simulink model "mpu6050 - Copy"  (R2017a)
settings: Solver=FixedStepDiscrete  StartTime=0.0  StopTime=inf  RelTol=1e-3
PostLoadFcn:
  | ChipSelect = 1;  % choose I2C comms
  | AddressAlt = 0;  % use default address
  | 
  | if AddressAlt == 1
  | % b1101001 (pin AD0 is logic high).
  | SlvAddr = uint8(bin2dec('1101001'));  % ADDR ALT = 1
  | else
  | % b1101000 (pin AD0 is logic low)
  | SlvAddr = uint8(bin2dec('1101000'));  % ADDR ALT = 0
  | end
  | SlvAddr = uint8(hex2dec('68'));
  | 
  | 
  | % 0x3B 59 ACCEL_XOUT[15:8]
  | % 0x3C 60 ACCEL_XOUT[7:0]
  | % 0x3D 61 ACCEL_YOUT[15:8]
  | % 0x3E 62 ACCEL_YOUT[7:0]
  | % 0x3F 63 ACCEL_ZOUT[15:8]
  | % 0x40 64 ACCEL_ZOUT[7:0]
  | 
  | AccelXRegAddr = uint8(hex2dec('3B'));
  | AccelYRegAddr = uint8(hex2dec('3D'));
  | AccelZRegAddr = uint8(hex2dec('3F'));
  | 
  | % 0x43 67 GYRO_XOUT[15:8]
  | % 0x44 68 GYRO_XOUT[7:0]
  | % 0x45 69 GYRO_YOUT[15:8]
  | % 0x46 70 GYRO_YOUT[7:0]
  | % 0x47 71 GYRO_ZOUT[15:8]
  | % 0x48 72 GYRO_ZOUT[7:0]
  | 
  | GyroXRegAddr = uint8(hex2dec('43'));
  | GyroYRegAddr = uint8(hex2dec('45'));
  | GyroZRegAddr = uint8(hex2dec('47'));
  | 
  | deviceAddr = fi(SlvAddr,0,7,0);
  | 
  | powerRegAddr = uint8(hex2dec('6B'));
  | powerRegData = bin2dec('10000001');
(part 1 of 4)
settings Model: DataTypeOverride=Off  Creator=skuznick  LastModifiedBy=mini
settings DataIOCC: SaveOutput=off  SaveTime=off
settings OptimizationCC: BlockReduction=off  ConditionallyExecuteInputs=off  DefaultParameterBehavior=Inlined
settings DebuggingCC: AlgebraicLoopMsg=error  SingleTaskRateTransMsg=error
settings HardwareCC: ProdBitPerPointer=32  ProdBitPerSizeT=32  ProdBitPerPtrDiffT=32  ProdLargestAtomicFloat=None  ProdIntDivRoundTo=Undefined  ProdEndianess=Unspecified  ProdWordSize=32  ProdHWDeviceType=ASIC/FPGA->ASIC/FPGA  ProdEqTarget=off
settings GRTTargetCC: ExtMode=on

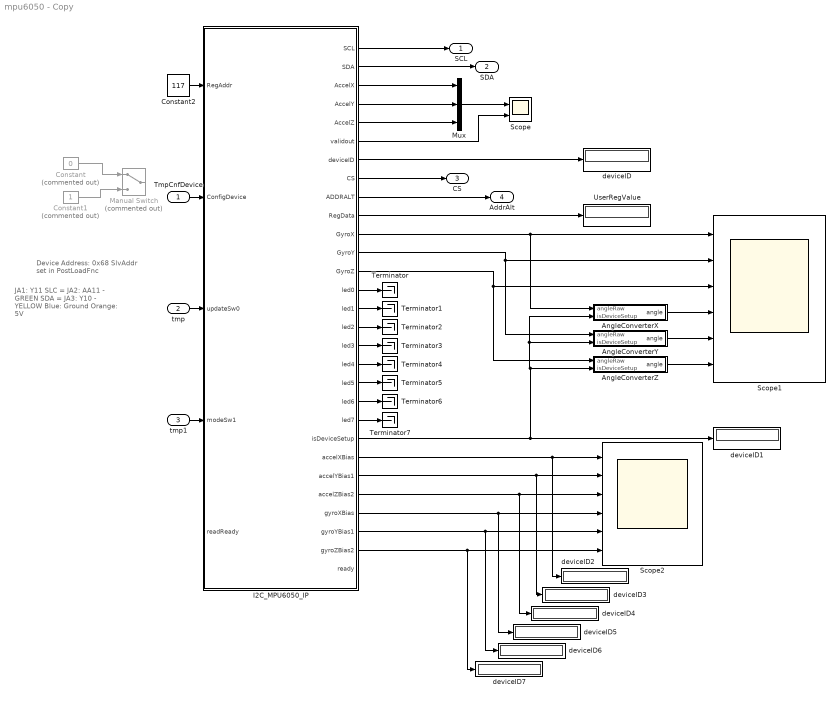
== system mpu6050 - Copy ==
  note: JA1: Y11
      | SLC = JA2: AA11 - GREEN
      | SDA = JA3: Y10  - YELLOW
      | Blue: Ground
      | Orange: 5V
  note: Device Address: 0x68
      | SlvAddr set in PostLoadFnc
  TmpCnfDevice : Inport  OutDataTypeStr=boolean
  tmp : Inport  Port=2  OutDataTypeStr=boolean
  tmp1 : Inport  Port=3  OutDataTypeStr=boolean
  AngleConverterX : Subsystem
  AngleConverterY : Subsystem
  AngleConverterZ : Subsystem
  Constant : Constant  Commented=on  Value=0  OutDataTypeStr=boolean  SampleTime=-1
  Constant1 : Constant  Commented=on  OutDataTypeStr=boolean  SampleTime=-1
  Constant2 : Constant  Value=117  OutDataTypeStr=uint8  SampleTime=-1
  I2C_MPU6050_IP : Subsystem  TreatAsAtomicUnit=on  SystemSampleTime=1/400e3
  Manual Switch : ManualSwitch  Commented=on
  Mux : Mux  Inputs=3
  Scope : Scope  NumInputPorts=2
  Scope1 : Scope  NumInputPorts=6
  Scope2 : Scope  NumInputPorts=6
  Terminator{,1..7} (8 alike) : Terminator
  UserRegValue : Display
  deviceID{,1..7} (8 alike) : Display
      deviceID2 settings: Decimation=5
      deviceID3 settings: Decimation=5
      deviceID4 settings: Decimation=5
      deviceID5 settings: Decimation=5
      deviceID6 settings: Decimation=5
      deviceID7 settings: Decimation=5
  SCL : Outport
  SDA : Outport  Port=2
  CS : Outport  Port=3
  AddrAlt : Outport  Port=4
  wires:
  I2C_MPU6050_IP/2(SDA) -> SDA/1
  I2C_MPU6050_IP/1(SCL) -> SCL/1
  I2C_MPU6050_IP/8(CS) -> CS/1
  I2C_MPU6050_IP/9(ADDRALT) -> AddrAlt/1
  I2C_MPU6050_IP/4(AccelY) -> Mux/2
  I2C_MPU6050_IP/3(AccelX) -> Mux/1
  I2C_MPU6050_IP/5(AccelZ) -> Mux/3
  I2C_MPU6050_IP/7(deviceID) -> deviceID/1
  I2C_MPU6050_IP/10(RegData) -> UserRegValue/1
  Mux/1 -> Scope/1
  Constant/1 -> Manual Switch/1
  Constant1/1 -> Manual Switch/2
  Constant2/1 -> I2C_MPU6050_IP/1(RegAddr)
  I2C_MPU6050_IP/13(GyroZ) -> AngleConverterZ/1(angleRaw), Scope1/3
  I2C_MPU6050_IP/11(GyroX) -> AngleConverterX/1(angleRaw), Scope1/1
  I2C_MPU6050_IP/12(GyroY) -> AngleConverterY/1(angleRaw), Scope1/2
  I2C_MPU6050_IP/6(validout) -> Scope/2
  TmpCnfDevice/1 -> I2C_MPU6050_IP/2(ConfigDevice)
  I2C_MPU6050_IP/14(led0) -> Terminator/1
  I2C_MPU6050_IP/15(led1) -> Terminator1/1
  I2C_MPU6050_IP/16(led2) -> Terminator2/1
  I2C_MPU6050_IP/17(led3) -> Terminator3/1
  I2C_MPU6050_IP/20(led6) -> Terminator6/1
  I2C_MPU6050_IP/21(led7) -> Terminator7/1
  I2C_MPU6050_IP/19(led5) -> Terminator5/1
  I2C_MPU6050_IP/18(led4) -> Terminator4/1
  tmp/1 -> I2C_MPU6050_IP/3(updateSw0)
  tmp1/1 -> I2C_MPU6050_IP/4(modeSw1)
  I2C_MPU6050_IP/22(isDeviceSetup) -> deviceID1/1, AngleConverterZ/2(isDeviceSetup), AngleConverterX/2(isDeviceSetup), AngleConverterY/2(isDeviceSetup)
  AngleConverterY/1(angle) -> Scope1/5
  AngleConverterZ/1(angle) -> Scope1/6
  AngleConverterX/1(angle) -> Scope1/4
  I2C_MPU6050_IP/23(accelXBias) -> deviceID2/1, Scope2/1
  I2C_MPU6050_IP/24(accelYBias1) -> deviceID3/1, Scope2/2
  I2C_MPU6050_IP/25(accelZBias2) -> deviceID4/1, Scope2/3
  I2C_MPU6050_IP/26(gyroXBias) -> deviceID5/1, Scope2/4
  I2C_MPU6050_IP/27(gyroYBias1) -> deviceID6/1, Scope2/5
  I2C_MPU6050_IP/28(gyroZBias2) -> deviceID7/1, Scope2/6

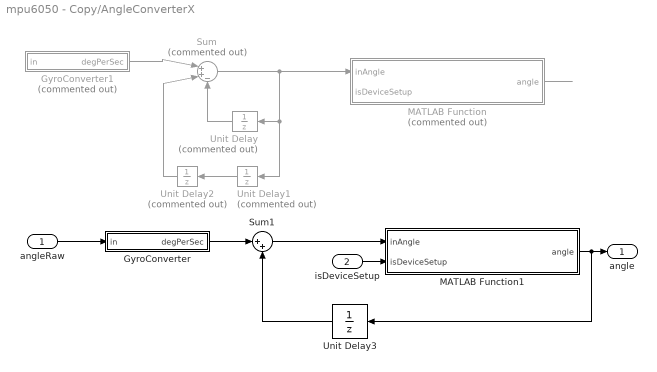
== system mpu6050 - Copy/AngleConverterX ==
  angleRaw : Inport  OutDataTypeStr=int16  Interpolate=off
  isDeviceSetup : Inport  Port=2  OutDataTypeStr=boolean  Interpolate=off
  GyroConverter : Subsystem
  GyroConverter1 : Subsystem  Commented=on
  MATLAB Function : MATLAB Function  Commented=on  TreatAsAtomicUnit=on
  MATLAB Function1 : MATLAB Function  TreatAsAtomicUnit=on
  Sum : Sum  Commented=on  Inputs=|++-  SaturateOnIntegerOverflow=off  InputSameDT=off  OutDataTypeStr=Inherit: Inherit via internal rule
  Sum1 : Sum  Inputs=|++  SaturateOnIntegerOverflow=off  InputSameDT=off  OutDataTypeStr=Inherit: Inherit via internal rule
  Unit Delay : UnitDelay  Commented=on  SampleTime=-1
  Unit Delay1 : UnitDelay  Commented=on  SampleTime=-1
  Unit Delay2 : UnitDelay  Commented=on  SampleTime=-1
  Unit Delay3 : UnitDelay  SampleTime=-1
  angle : Outport  OutDataTypeStr=double
  wires:
  Sum/1 -> Unit Delay1/1, Unit Delay/1, MATLAB Function/1(inAngle)
  GyroConverter1/1(degPerSec) -> Sum/1
  Unit Delay/1 -> Sum/3
  Unit Delay1/1 -> Unit Delay2/1
  Unit Delay2/1 -> Sum/2
  MATLAB Function/1(angle) -> ?
  ? -> MATLAB Function/2(isDeviceSetup)
  MATLAB Function1/1(angle) -> Unit Delay3/1, angle/1
  angleRaw/1 -> GyroConverter/1(in)
  isDeviceSetup/1 -> MATLAB Function1/2(isDeviceSetup)
  GyroConverter/1(degPerSec) -> Sum1/1
  Sum1/1 -> MATLAB Function1/1(inAngle)
  Unit Delay3/1 -> Sum1/2

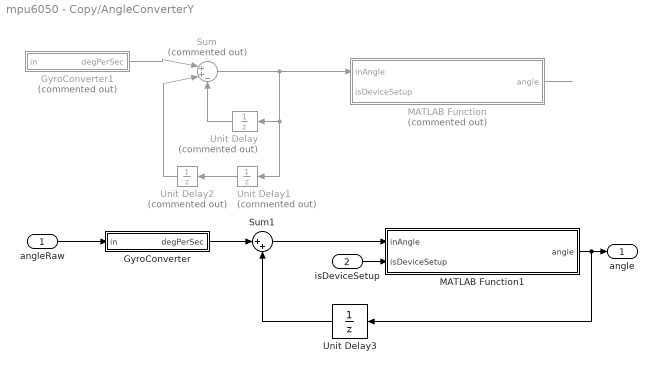
== system mpu6050 - Copy/AngleConverterY ==
  angleRaw : Inport  OutDataTypeStr=int16  Interpolate=off
  isDeviceSetup : Inport  Port=2  OutDataTypeStr=boolean  Interpolate=off
  GyroConverter : Subsystem
  GyroConverter1 : Subsystem  Commented=on
  MATLAB Function : MATLAB Function  Commented=on  TreatAsAtomicUnit=on
  MATLAB Function1 : MATLAB Function  TreatAsAtomicUnit=on
  Sum : Sum  Commented=on  Inputs=|++-  SaturateOnIntegerOverflow=off  InputSameDT=off  OutDataTypeStr=Inherit: Inherit via internal rule
  Sum1 : Sum  Inputs=|++  SaturateOnIntegerOverflow=off  InputSameDT=off  OutDataTypeStr=Inherit: Inherit via internal rule
  Unit Delay : UnitDelay  Commented=on  SampleTime=-1
  Unit Delay1 : UnitDelay  Commented=on  SampleTime=-1
  Unit Delay2 : UnitDelay  Commented=on  SampleTime=-1
  Unit Delay3 : UnitDelay  SampleTime=-1
  angle : Outport  OutDataTypeStr=double
  wires:
  Sum/1 -> Unit Delay1/1, Unit Delay/1, MATLAB Function/1(inAngle)
  GyroConverter1/1(degPerSec) -> Sum/1
  Unit Delay/1 -> Sum/3
  Unit Delay1/1 -> Unit Delay2/1
  Unit Delay2/1 -> Sum/2
  MATLAB Function/1(angle) -> ?
  ? -> MATLAB Function/2(isDeviceSetup)
  MATLAB Function1/1(angle) -> Unit Delay3/1, angle/1
  angleRaw/1 -> GyroConverter/1(in)
  isDeviceSetup/1 -> MATLAB Function1/2(isDeviceSetup)
  GyroConverter/1(degPerSec) -> Sum1/1
  Sum1/1 -> MATLAB Function1/1(inAngle)
  Unit Delay3/1 -> Sum1/2

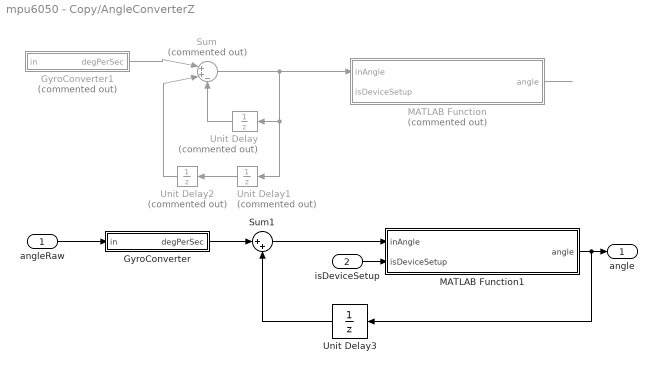
== system mpu6050 - Copy/AngleConverterZ ==
  angleRaw : Inport  OutDataTypeStr=int16  Interpolate=off
  isDeviceSetup : Inport  Port=2  OutDataTypeStr=boolean  Interpolate=off
  GyroConverter : Subsystem
  GyroConverter1 : Subsystem  Commented=on
  MATLAB Function : MATLAB Function  Commented=on  TreatAsAtomicUnit=on
  MATLAB Function1 : MATLAB Function  TreatAsAtomicUnit=on
  Sum : Sum  Commented=on  Inputs=|++-  SaturateOnIntegerOverflow=off  InputSameDT=off  OutDataTypeStr=Inherit: Inherit via internal rule
  Sum1 : Sum  Inputs=|++  SaturateOnIntegerOverflow=off  InputSameDT=off  OutDataTypeStr=Inherit: Inherit via internal rule
  Unit Delay : UnitDelay  Commented=on  SampleTime=-1
  Unit Delay1 : UnitDelay  Commented=on  SampleTime=-1
  Unit Delay2 : UnitDelay  Commented=on  SampleTime=-1
  Unit Delay3 : UnitDelay  SampleTime=-1
  angle : Outport  OutDataTypeStr=double
  wires:
  Sum/1 -> Unit Delay1/1, Unit Delay/1, MATLAB Function/1(inAngle)
  GyroConverter1/1(degPerSec) -> Sum/1
  Unit Delay/1 -> Sum/3
  Unit Delay1/1 -> Unit Delay2/1
  Unit Delay2/1 -> Sum/2
  MATLAB Function/1(angle) -> ?
  ? -> MATLAB Function/2(isDeviceSetup)
  MATLAB Function1/1(angle) -> Unit Delay3/1, angle/1
  angleRaw/1 -> GyroConverter/1(in)
  isDeviceSetup/1 -> MATLAB Function1/2(isDeviceSetup)
  GyroConverter/1(degPerSec) -> Sum1/1
  Sum1/1 -> MATLAB Function1/1(inAngle)
  Unit Delay3/1 -> Sum1/2

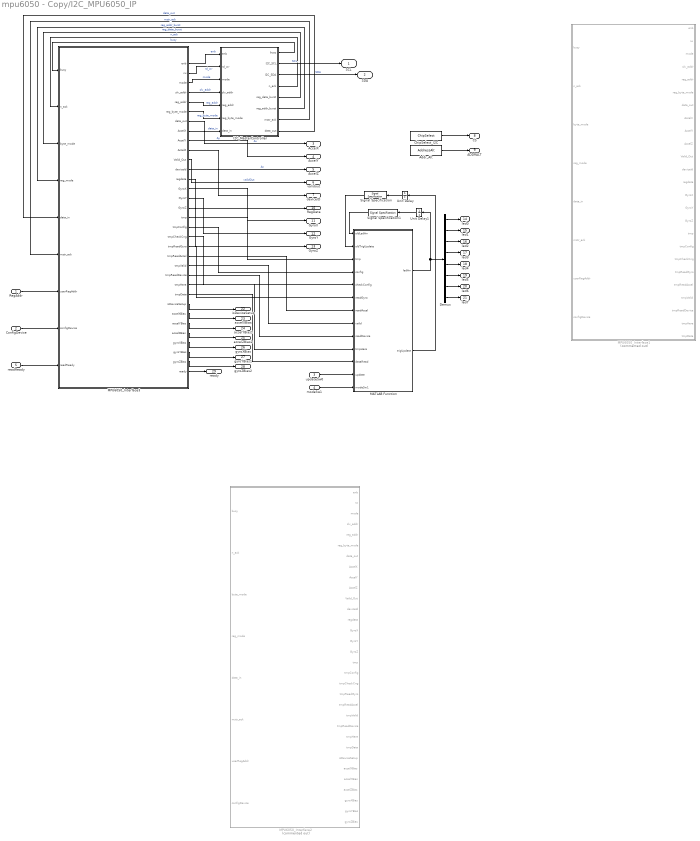
== system mpu6050 - Copy/I2C_MPU6050_IP ==
  RegAddr : Inport
  ConfigDevice : Inport  Port=2
  updateSw0 : Inport  Port=3  OutDataTypeStr=boolean
  modeSw1 : Inport  Port=4  OutDataTypeStr=boolean
  readReady : Inport  Port=5
  Addr_Alt : Constant  Value=AddressAlt  OutDataTypeStr=boolean  SampleTime=-1
  ChipSelect_I2C : Constant  Value=ChipSelect  OutDataTypeStr=boolean  SampleTime=-1
  Demux : Demux  Outputs=8
  I2C_MasterController : Subsystem
  MATLAB Function : MATLAB Function  TreatAsAtomicUnit=on
  MPU6050_Interface1 : Stateflow chart  Commented=on  TreatAsAtomicUnit=on
  MPU6050_Interface2 : Stateflow chart  Commented=on  TreatAsAtomicUnit=on
  MPU6050_Interface3 : Stateflow chart  TreatAsAtomicUnit=on
  Signal Specification : SignalSpecification  OutDataTypeStr=boolean
  Signal Specification1 : SignalSpecification  OutDataTypeStr=boolean  Dimensions=[1 8]
  Unit Delay : UnitDelay  SampleTime=-1
  Unit Delay1 : UnitDelay  SampleTime=-1
  SCL : Outport
  SDA : Outport  Port=2
  AccelX : Outport  Port=3
  AccelY : Outport  Port=4
  AccelZ : Outport  Port=5
  validout : Outport  Port=6
  deviceID : Outport  Port=7
  CS : Outport  Port=8
  ADDRALT : Outport  Port=9
  RegData : Outport  Port=10
  GyroX : Outport  Port=11
  GyroY : Outport  Port=12
  GyroZ : Outport  Port=13
  led0 : Outport  Port=14  OutDataTypeStr=boolean
  led1 : Outport  Port=15  OutDataTypeStr=boolean
  led2 : Outport  Port=16  OutDataTypeStr=boolean
  led3 : Outport  Port=17  OutDataTypeStr=boolean
  led4 : Outport  Port=18  OutDataTypeStr=boolean
  led5 : Outport  Port=19  OutDataTypeStr=boolean
  led6 : Outport  Port=20  OutDataTypeStr=boolean
  led7 : Outport  Port=21  OutDataTypeStr=boolean
  isDeviceSetup : Outport  Port=22  OutDataTypeStr=boolean
  accelXBias : Outport  Port=23
  accelYBias1 : Outport  Port=24
  accelZBias2 : Outport  Port=25
  gyroXBias : Outport  Port=26
  gyroYBias1 : Outport  Port=27
  gyroZBias2 : Outport  Port=28
  ready : Outport  Port=29  OutDataTypeStr=boolean
  wires:
  MPU6050_Interface3/7(data_out) -> I2C_MasterController/7(data_in)  "data_in"
  I2C_MasterController/8(data_out) -> MPU6050_Interface3/5(data_in)  "data_out"
  I2C_MasterController/7(mstr_ack) -> MPU6050_Interface3/6(mstr_ack)  "mstr_ack"
  I2C_MasterController/4(n_ack) -> MPU6050_Interface3/2(n_ack)  "n_ack"
  I2C_MasterController/5(reg_data_burst) -> MPU6050_Interface3/3(byte_mode)  "reg_data_burst"
  I2C_MasterController/6(reg_addr_burst) -> MPU6050_Interface3/4(reg_mode)  "reg_addr_burst"
  I2C_MasterController/1(busy) -> MPU6050_Interface3/1(busy)  "busy"
  I2C_MasterController/3(I2C_SDA) -> SDA/1  "SDA"
  I2C_MasterController/2(I2C_SCL) -> SCL/1  "SCL"
  MPU6050_Interface3/6(reg_byte_mode) -> I2C_MasterController/6(reg_byte_mode)  "reg_byte_mode"
  MPU6050_Interface3/5(reg_addr) -> I2C_MasterController/5(reg_addr)  "reg_addr"
  MPU6050_Interface3/4(slv_addr) -> I2C_MasterController/4(slv_addr)  "slv_addr"
  MPU6050_Interface3/3(mode) -> I2C_MasterController/3(mode)  "mode"
  MPU6050_Interface3/2(rw) -> I2C_MasterController/2(rd_wr)  "rd_wr"
  MPU6050_Interface3/1(enb) -> I2C_MasterController/1(enb)  "enb"
  ChipSelect_I2C/1 -> CS/1
  Addr_Alt/1 -> ADDRALT/1
  MPU6050_Interface3/9(AccelY) -> AccelY/1  "Ay"
  MPU6050_Interface3/10(AccelZ) -> AccelZ/1  "Az"
  MPU6050_Interface3/11(Valid_Out) -> validout/1  "validOut"
  MPU6050_Interface3/8(AccelX) -> AccelX/1  "Ax"
  MPU6050_Interface3/12(deviceId) -> deviceID/1
  MPU6050_Interface3/13(regdata) -> RegData/1
  RegAddr/1 -> MPU6050_Interface3/7(userRegAddr)
  MPU6050_Interface3/14(GyroX) -> GyroX/1
  MPU6050_Interface3/15(GyroY) -> GyroY/1
  MPU6050_Interface3/16(GyroZ) -> GyroZ/1
  ConfigDevice/1 -> MPU6050_Interface3/8(configDevice)
  MPU6050_Interface3/17(tmp) -> MATLAB Function/3(tmp)
  MPU6050_Interface3/18(tmpConfig) -> MATLAB Function/4(config)
  MPU6050_Interface3/19(tmpCheckCng) -> MATLAB Function/5(checkConfig)
  MPU6050_Interface3/20(tmpReadGyro) -> MATLAB Function/6(readGyro)
  MPU6050_Interface3/21(tmpReadAccel) -> MATLAB Function/7(readAccel)
  MPU6050_Interface3/22(tmpValid) -> MATLAB Function/8(valid)
  MPU6050_Interface3/23(tmpReadDevice) -> MATLAB Function/9(readDevice)
  MATLAB Function/1(ledArr) -> Unit Delay1/1, Demux/1
  MATLAB Function/2(trigUpdate) -> Unit Delay/1
  Demux/1 -> led0/1
  Demux/8 -> led7/1
  Demux/7 -> led6/1
  Demux/6 -> led5/1
  Demux/5 -> led4/1
  Demux/4 -> led3/1
  Demux/3 -> led2/1
  Demux/2 -> led1/1
  updateSw0/1 -> MATLAB Function/12(update)
  modeSw1/1 -> MATLAB Function/13(modeSw1)
  Unit Delay/1 -> Signal Specification/1
  Signal Specification/1 -> MATLAB Function/2(oldTrigUpdate)
  Unit Delay1/1 -> Signal Specification1/1
  Signal Specification1/1 -> MATLAB Function/1(oldLedArr)
  MPU6050_Interface3/24(tmpHere) -> MATLAB Function/10(tmpHere)
  MPU6050_Interface3/25(tmpData) -> MATLAB Function/11(dataRead)
  MPU6050_Interface3/26(isDeviceSetup) -> isDeviceSetup/1
  MPU6050_Interface3/27(accelXBias) -> accelXBias/1
  MPU6050_Interface3/29(accelZBias) -> accelZBias2/1
  MPU6050_Interface3/28(accelYBias) -> accelYBias1/1
  MPU6050_Interface3/30(gyroXBias) -> gyroXBias/1
  MPU6050_Interface3/31(gyroYBias) -> gyroYBias1/1
  MPU6050_Interface3/32(gyroZBias) -> gyroZBias2/1
  MPU6050_Interface3/33(ready) -> ready/1
  readReady/1 -> MPU6050_Interface3/9(readReady)

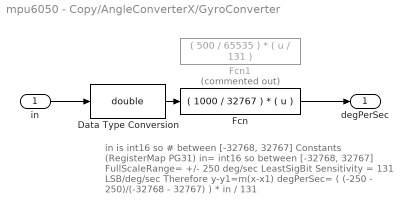
== system mpu6050 - Copy/AngleConverterX/GyroConverter ==
  note: in is int16 so # between [-32768, 32767]
      | Constants (RegisterMap PG31)
      | in= int16 so between [-32768, 32767]
      | FullScaleRange= +/- 250 deg/sec
      | LeastSigBit Sensitivity = 131 LSB/deg/sec
      | Therefore
      | y-y1=m(x-x1)
      | degPerSec= ( (-250 - 250)/(-32768 - 32767) ) * in / 131
  in : Inport  OutDataTypeStr=int16  Interpolate=off
  Data Type Conversion : DataTypeConversion  OutDataTypeStr=double  SaturateOnIntegerOverflow=off  RndMeth=Floor
  Fcn : Fcn  Expr=( 1000 / 32767 ) * ( u )
  Fcn1 : Fcn  Commented=on  Expr=( 500 / 65535 ) * ( u / 131 )
  degPerSec : Outport  OutDataTypeStr=double
  wires:
  Fcn/1 -> degPerSec/1
  in/1 -> Data Type Conversion/1
  Data Type Conversion/1 -> Fcn/1

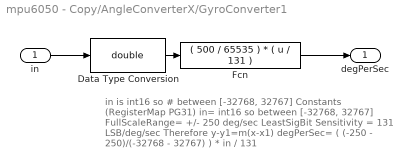
== system mpu6050 - Copy/AngleConverterX/GyroConverter1 ==
  note: in is int16 so # between [-32768, 32767]
      | Constants (RegisterMap PG31)
      | in= int16 so between [-32768, 32767]
      | FullScaleRange= +/- 250 deg/sec
      | LeastSigBit Sensitivity = 131 LSB/deg/sec
      | Therefore
      | y-y1=m(x-x1)
      | degPerSec= ( (-250 - 250)/(-32768 - 32767) ) * in / 131
  in : Inport  OutDataTypeStr=int16  Interpolate=off
  Data Type Conversion : DataTypeConversion  OutDataTypeStr=double  SaturateOnIntegerOverflow=off  RndMeth=Floor
  Fcn : Fcn  Expr=( 500 / 65535 ) * ( u / 131 )
  degPerSec : Outport  OutDataTypeStr=double
  wires:
  Data Type Conversion/1 -> Fcn/1
  in/1 -> Data Type Conversion/1
  Fcn/1 -> degPerSec/1

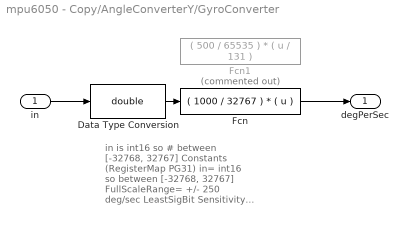
== system mpu6050 - Copy/AngleConverterY/GyroConverter ==
  note: in is int16 so # between [-32768, 32767]
      | Constants (RegisterMap PG31)
      | in= int16 so between [-32768, 32767]
      | FullScaleRange= +/- 250 deg/sec
      | LeastSigBit Sensitivity = 131 LSB/deg/sec
      | Therefore
      | y-y1=m(x-x1)
      | degPerSec= ( (-250 - 250)/(-32768 - 32767) ) * in / 131
  in : Inport  OutDataTypeStr=int16  Interpolate=off
  Data Type Conversion : DataTypeConversion  OutDataTypeStr=double  SaturateOnIntegerOverflow=off  RndMeth=Floor
  Fcn : Fcn  Expr=( 1000 / 32767 ) * ( u )
  Fcn1 : Fcn  Commented=on  Expr=( 500 / 65535 ) * ( u / 131 )
  degPerSec : Outport  OutDataTypeStr=double
  wires:
  Fcn/1 -> degPerSec/1
  in/1 -> Data Type Conversion/1
  Data Type Conversion/1 -> Fcn/1

== system mpu6050 - Copy/AngleConverterY/GyroConverter1 ==
  note: in is int16 so # between [-32768, 32767]
      | Constants (RegisterMap PG31)
      | in= int16 so between [-32768, 32767]
      | FullScaleRange= +/- 250 deg/sec
      | LeastSigBit Sensitivity = 131 LSB/deg/sec
      | Therefore
      | y-y1=m(x-x1)
      | degPerSec= ( (-250 - 250)/(-32768 - 32767) ) * in / 131
  in : Inport  OutDataTypeStr=int16  Interpolate=off
  Data Type Conversion : DataTypeConversion  OutDataTypeStr=double  SaturateOnIntegerOverflow=off  RndMeth=Floor
  Fcn : Fcn  Expr=( 500 / 65535 ) * ( u / 131 )
  degPerSec : Outport  OutDataTypeStr=double
  wires:
  Data Type Conversion/1 -> Fcn/1
  in/1 -> Data Type Conversion/1
  Fcn/1 -> degPerSec/1

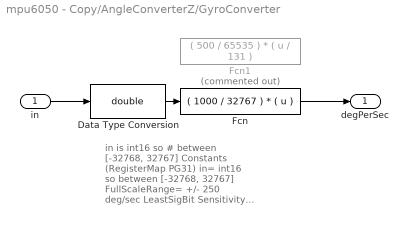
== system mpu6050 - Copy/AngleConverterZ/GyroConverter ==
  note: in is int16 so # between [-32768, 32767]
      | Constants (RegisterMap PG31)
      | in= int16 so between [-32768, 32767]
      | FullScaleRange= +/- 250 deg/sec
      | LeastSigBit Sensitivity = 131 LSB/deg/sec
      | Therefore
      | y-y1=m(x-x1)
      | degPerSec= ( (-250 - 250)/(-32768 - 32767) ) * in / 131
  in : Inport  OutDataTypeStr=int16  Interpolate=off
  Data Type Conversion : DataTypeConversion  OutDataTypeStr=double  SaturateOnIntegerOverflow=off  RndMeth=Floor
  Fcn : Fcn  Expr=( 1000 / 32767 ) * ( u )
  Fcn1 : Fcn  Commented=on  Expr=( 500 / 65535 ) * ( u / 131 )
  degPerSec : Outport  OutDataTypeStr=double
  wires:
  Fcn/1 -> degPerSec/1
  in/1 -> Data Type Conversion/1
  Data Type Conversion/1 -> Fcn/1

== system mpu6050 - Copy/AngleConverterZ/GyroConverter1 ==
  note: in is int16 so # between [-32768, 32767]
      | Constants (RegisterMap PG31)
      | in= int16 so between [-32768, 32767]
      | FullScaleRange= +/- 250 deg/sec
      | LeastSigBit Sensitivity = 131 LSB/deg/sec
      | Therefore
      | y-y1=m(x-x1)
      | degPerSec= ( (-250 - 250)/(-32768 - 32767) ) * in / 131
  in : Inport  OutDataTypeStr=int16  Interpolate=off
  Data Type Conversion : DataTypeConversion  OutDataTypeStr=double  SaturateOnIntegerOverflow=off  RndMeth=Floor
  Fcn : Fcn  Expr=( 500 / 65535 ) * ( u / 131 )
  degPerSec : Outport  OutDataTypeStr=double
  wires:
  Data Type Conversion/1 -> Fcn/1
  in/1 -> Data Type Conversion/1
  Fcn/1 -> degPerSec/1

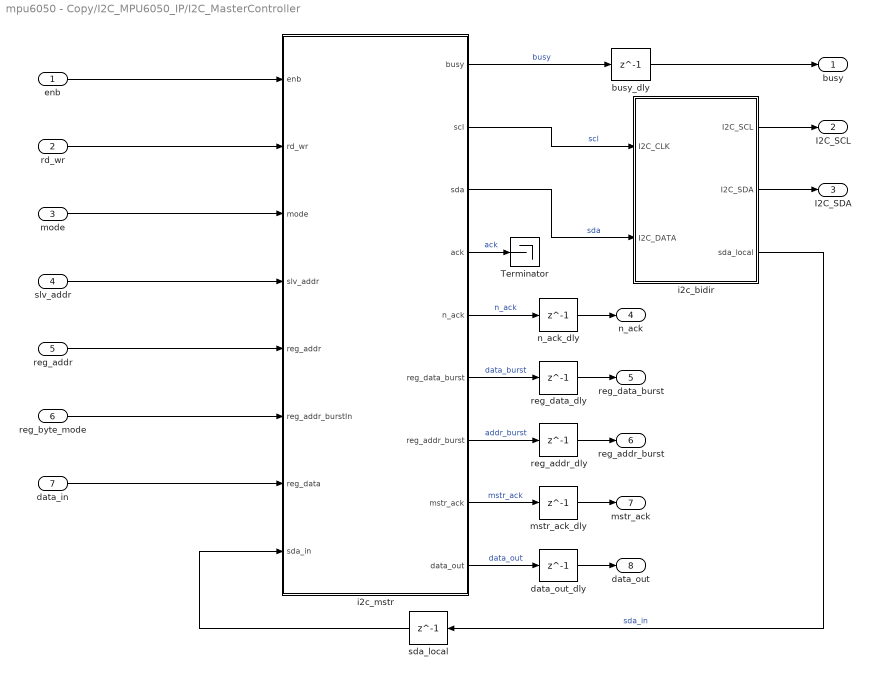
== system mpu6050 - Copy/I2C_MPU6050_IP/I2C_MasterController ==
  enb : Inport
  rd_wr : Inport  Port=2
  mode : Inport  Port=3
  slv_addr : Inport  Port=4
  reg_addr : Inport  Port=5
  reg_byte_mode : Inport  Port=6
  data_in : Inport  Port=7
  Terminator : Terminator
  busy_dly : Delay  DelayLength=1
  data_out_dly : Delay  DelayLength=1
  i2c_bidir : Subsystem  TreatAsAtomicUnit=on
  i2c_mstr : Stateflow chart  TreatAsAtomicUnit=on
  mstr_ack_dly : Delay  DelayLength=1
  n_ack_dly : Delay  DelayLength=1
  reg_addr_dly : Delay  DelayLength=1
  reg_data_dly : Delay  DelayLength=1
  sda_local : Delay  DelayLength=1
  busy : Outport
  I2C_SCL : Outport  Port=2
  I2C_SDA : Outport  Port=3
  n_ack : Outport  Port=4
  reg_data_burst : Outport  Port=5
  reg_addr_burst : Outport  Port=6
  mstr_ack : Outport  Port=7
  data_out : Outport  Port=8
  wires:
  data_out_dly/1 -> data_out/1
  mstr_ack_dly/1 -> mstr_ack/1
  i2c_mstr/9(data_out) -> data_out_dly/1  "data_out"
  i2c_mstr/8(mstr_ack) -> mstr_ack_dly/1  "mstr_ack"
  busy_dly/1 -> busy/1
  n_ack_dly/1 -> n_ack/1
  reg_data_dly/1 -> reg_data_burst/1
  reg_addr_dly/1 -> reg_addr_burst/1
  i2c_mstr/1(busy) -> busy_dly/1  "busy"
  rd_wr/1 -> i2c_mstr/2(rd_wr)
  mode/1 -> i2c_mstr/3(mode)
  data_in/1 -> i2c_mstr/7(reg_data)
  enb/1 -> i2c_mstr/1(enb)
  slv_addr/1 -> i2c_mstr/4(slv_addr)
  reg_byte_mode/1 -> i2c_mstr/6(reg_addr_burstIn)
  reg_addr/1 -> i2c_mstr/5(reg_addr)
  i2c_bidir/1(I2C_SCL) -> I2C_SCL/1
  i2c_bidir/2(I2C_SDA) -> I2C_SDA/1
  i2c_mstr/4(ack) -> Terminator/1  "ack"
  i2c_mstr/2(scl) -> i2c_bidir/1(I2C_CLK)  "scl"
  i2c_bidir/3(sda_local) -> sda_local/1  "sda_in"
  sda_local/1 -> i2c_mstr/8(sda_in)
  i2c_mstr/3(sda) -> i2c_bidir/2(I2C_DATA)  "sda"
  i2c_mstr/5(n_ack) -> n_ack_dly/1  "n_ack"
  i2c_mstr/6(reg_data_burst) -> reg_data_dly/1  "data_burst"
  i2c_mstr/7(reg_addr_burst) -> reg_addr_dly/1  "addr_burst"

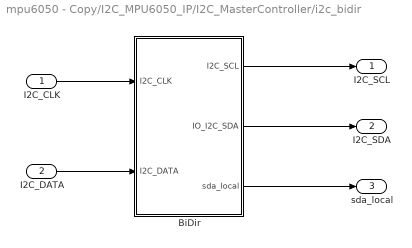
== system mpu6050 - Copy/I2C_MPU6050_IP/I2C_MasterController/i2c_bidir ==
  I2C_CLK : Inport
  I2C_DATA : Inport  Port=2
  BiDir : Subsystem  TreatAsAtomicUnit=on
  I2C_SCL : Outport
  I2C_SDA : Outport  Port=2
  sda_local : Outport  Port=3
  wires:
  BiDir/2(IO_I2C_SDA) -> I2C_SDA/1
  I2C_CLK/1 -> BiDir/1(I2C_CLK)
  I2C_DATA/1 -> BiDir/2(I2C_DATA)
  BiDir/1("I2C_SCL ") -> I2C_SCL/1
  BiDir/3(sda_local) -> sda_local/1

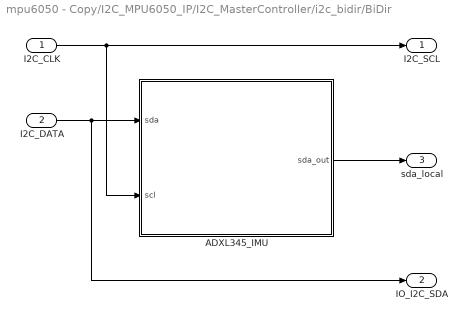
== system mpu6050 - Copy/I2C_MPU6050_IP/I2C_MasterController/i2c_bidir/BiDir ==
  I2C_CLK : Inport  OutDataTypeStr=boolean
  I2C_DATA : Inport  Port=2  OutDataTypeStr=boolean
  ADXL345_IMU : Stateflow chart  TreatAsAtomicUnit=on
  "I2C_SCL " : Outport  OutDataTypeStr=boolean
  IO_I2C_SDA : Outport  Port=2  OutDataTypeStr=boolean
  sda_local : Outport  Port=3  OutDataTypeStr=boolean
  wires:
  ADXL345_IMU/1(sda_out) -> sda_local/1
  I2C_CLK/1 -> "I2C_SCL "/1, ADXL345_IMU/2(scl)
  I2C_DATA/1 -> IO_I2C_SDA/1, ADXL345_IMU/1(sda)
